simulink model "SG__MDL_IO104_setup"  (R2022a)
settings: Solver=FixedStepAuto  StartTime=0.0  StopTime=Inf  RelTol=1e-3  EnableMultiTasking=on
model workspace (MAT data in the model file):
  a = 0.28
  ff = 1200
  fi = 150
  tmax = 40
undefined symbols (not defined in the file or in its folder): Ended, Single
libraries: simulink x4, dspfdesign x3, speedgoatlib_IO104 x3, hdlsllib x2, slrealtimeloglib x1, dspsrcs4 x1
settings Model: SimulationMode=external  Creator=padlewsk  LastModifiedBy=padlewsk
settings SolverCC: ConcurrentTasks=on  AlgebraicLoopSolver=TrustRegion  PositivePriorityOrder=on  AutoInsertRateTranBlk=on
settings DataIOCC: SaveFormat=StructureWithTime
settings OptimizationCC: BlockReduction=off  OptimizeBlockIOStorage=off
settings DebuggingCC: TasksWithSamePriorityMsg=none  UnconnectedInputMsg=warning  UnconnectedOutputMsg=warning  UnconnectedLineMsg=warning
settings HardwareCC: ProdBitPerLong=64  ProdLongLongMode=on  ProdHWDeviceType=Intel->x86-64 (Linux 64)
settings RTWCC: Description=Simulink Real-Time  SystemTargetFile=slrealtime.tlc  TemplateMakefile=slrealtime_default_tmf  Toolchain=Simulink Real-Time Toolchain  BuildConfiguration=Faster Runs  CodeExecutionProfiling=on  TargetLang=C++

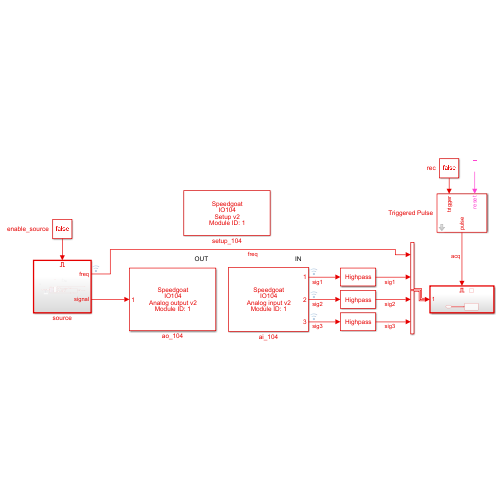
[thumbnail: Simulink's stored preview of the top-level diagram]
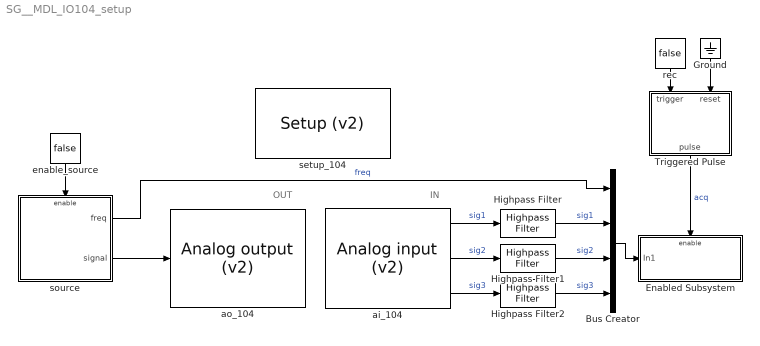
== system SG__MDL_IO104_setup ==
  note: IN
  note: OUT
  Bus Creator : BusCreator  Inputs=4
  Enabled Subsystem : Subsystem  TreatAsAtomicUnit=on
  Ground : Ground
  Highpass Filter : dspfdesign/Highpass Filter  FilterType=IIR  DesignForMinimumOrder=off  FilterOrder=4  StopbandFrequency=1  PassbandFrequency=5  StopbandAttenuation=40  PassbandRipple=0.5  InheritSampleRate=off  SampleRate=44100  SimulateUsing=Interpreted execution  roundingMode=Floor  coeffsDataTypeStr=fixdt(1,16)
  Highpass Filter1 : dspfdesign/Highpass Filter  FilterType=IIR  DesignForMinimumOrder=off  FilterOrder=4  StopbandFrequency=1  PassbandFrequency=5  StopbandAttenuation=40  PassbandRipple=0.5  InheritSampleRate=off  SampleRate=44100  SimulateUsing=Interpreted execution  roundingMode=Floor  coeffsDataTypeStr=fixdt(1,16)
  Highpass Filter2 : dspfdesign/Highpass Filter  FilterType=IIR  DesignForMinimumOrder=off  FilterOrder=4  StopbandFrequency=1  PassbandFrequency=5  StopbandAttenuation=40  PassbandRipple=0.5  InheritSampleRate=off  SampleRate=44100  SimulateUsing=Interpreted execution  roundingMode=Floor  coeffsDataTypeStr=fixdt(1,16)
  Triggered Pulse : Subsystem  mask(Triggered Pulse){N=4}
      mask prompts: N "Length (N samples)"
      mask help: Generates a single pulse of N samples length
  ai_104 : speedgoatlib_IO104/Analog input (v2)   parModuleId=1  parTs=0.0001  parPciSlot=-1  parAdChannels=[1,2,3]  parAdChannelsSorted=[1,2,3]  parAdRange1=+-2.5V  parAdRange2=+-2.5V  parAdCoupling=Single-Ended  parAdFrameSize=1  parAdUseTrigger=off  parAdClockInitiator=Initiator  parAdSampleTime=9.920634921e-07  parTriggerInitiator=Target  parTriggerRate=4.161015625e-01
      settings: SourceProductName=Simulink Real-Time: Speedgoat I/O Blockset
  ao_104 : speedgoatlib_IO104/Analog output (v2)   parModuleId=1  parTs=0.0001  parPciSlot=-1  parDaChannels=1  parDaChannelsSorted=1  parDaInitValue=0  parDaReset=1  parDaRange=+-2.5V  parDaFrameSize=1  parDaUseTrigger=off  parDaClockInitiator=Initiator  parDaSampleTime=9.920634921e-07  parTriggerInitiator=Target  parTriggerRate=4.161015625e-01  parAdBlockPresent=1
      settings: SourceProductName=Simulink Real-Time: Speedgoat I/O Blockset
  enable_source : Constant  Value=false  SampleTime=-1
  rec : Constant  Value=false  SampleTime=-1
  setup_104 : speedgoatlib_IO104/Setup (v2)   parPciSlot=-1  parModuleId=1  parTriggerInitiator=Target  parTriggerRate=4.161015625e-01  parCalibrate=off  parAdChannels=[1:3]  parAdRange1=+-2.5V  parAdRange2=+-2.5V  parAdCoupling=Single-Ended  parAdUseTrigger=off  parAdFrameSize=1  parAdClockInitiator=Initiator  parAdSampleTime=9.920634921e-07  parDaChannels=[1]  parDaChannelsSorted=1  parDaInitValue=[0]  parDaReset=[1]  parDaRange=+-2.5V  parDaUseTrigger=off  parDaFrameSize=1  parDaClockInitiator=Initiator  parDaSampleTime=9.920634921e-07  parDioByte0Dir=Outputs  parDioByte1Dir=Inputs  parDoChannels=[1:4]  parDoInitValues=[0]  parDoReset=[1]  parDiChannels=[13:16]
      settings: SourceProductName=Simulink Real-Time: Speedgoat I/O Blockset
  source : Subsystem  TreatAsAtomicUnit=on
  wires:
  enable_source/1 -> source/Enable
  source/2(signal) -> ao_104/1
  Triggered Pulse/1(pulse) -> Enabled Subsystem/Enable  "acq"
  Ground/1 -> Triggered Pulse/2(reset)
  rec/1 -> Triggered Pulse/1(trigger)
  Bus Creator/1 -> Enabled Subsystem/1(In1)
  source/1(freq) -> Bus Creator/1  "freq"
  ai_104/1 -> Highpass Filter/1  "sig1"
  ai_104/2 -> Highpass Filter1/1  "sig2"
  ai_104/3 -> Highpass Filter2/1  "sig3"
  Highpass Filter/1 -> Bus Creator/2  "sig1"
  Highpass Filter1/1 -> Bus Creator/3  "sig2"
  Highpass Filter2/1 -> Bus Creator/4  "sig3"

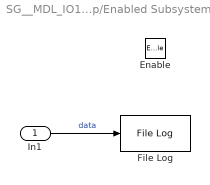
== system SG__MDL_IO104_setup/Enabled Subsystem ==
  In1 : Inport
  Enable : EnablePort
  File Log : slrealtimeloglib/File Log  decimation=1  inputProcessing=Elements as channels (sample based)
      settings: SourceProductBaseCode=XP
  wires:
  In1/1 -> File Log/1  "data"

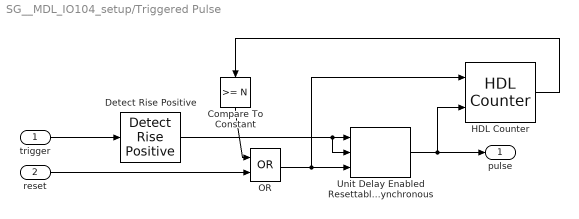
== system SG__MDL_IO104_setup/Triggered Pulse ==
  trigger : Inport
  reset : Inport  Port=2
  Compare To Constant : simulink/Logic and Bit Operations/Compare To Constant  relop=>=  const=N  OutDataTypeStr=boolean
  Detect Rise Positive : simulink/Logic and Bit Operations/Detect Rise Positive  vinit=0  OutDataTypeStr=boolean
  HDL Counter : hdlsllib/Sources/HDL Counter  CountType=Free running  CountInit=1  CountStep=1  CountMax=25  CountFromType=Initial value  CountFrom=1  CountResetPort=on  CountLoadPort=off  CountEnbPort=on  CountDirPort=off  CountHitOutputPort=off  CountDataType=Unsigned  CountWordLen=32  CountFracLen=0  CountSampTime=1
  OR : Logic  Operator=OR  AllPortsSameDT=off  OutDataTypeStr=boolean
  Unit Delay Enabled Resettable Synchronous : hdlsllib/Discrete/Unit Delay Enabled Resettable Synchronous  InitialCondition=0.0  SampleTime=-1
      settings: SourceProductBaseCode=SL
  pulse : Outport  VectorParamsAs1DForOutWhenUnconnected=off
  wires:
  OR/1 -> Unit Delay Enabled Resettable Synchronous/3, HDL Counter/1
  trigger/1 -> Detect Rise Positive/1
  Unit Delay Enabled Resettable Synchronous/1 -> HDL Counter/2, pulse/1
  Compare To Constant/1 -> OR/1
  reset/1 -> OR/2
  Detect Rise Positive/1 -> Unit Delay Enabled Resettable Synchronous/1, Unit Delay Enabled Resettable Synchronous/2
  HDL Counter/1 -> Compare To Constant/1

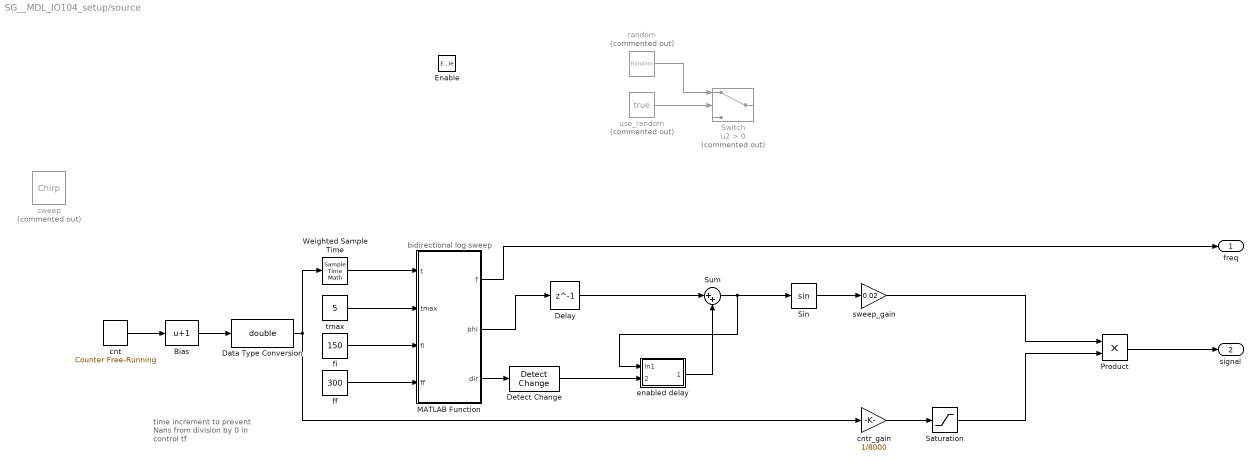
== system SG__MDL_IO104_setup/source ==
  note: bidirectional log sweep
  note: time increment to prevent Nans from division by 0 in control tf
  Enable : EnablePort  StatesWhenEnabling=reset
  Bias : Bias  Bias=1  SaturateOnIntegerOverflow=off
  Data Type Conversion : DataTypeConversion  OutDataTypeStr=double  SaturateOnIntegerOverflow=off  RndMeth=Floor
  Delay : Delay  DelayLength=1
  Detect Change : simulink/Logic and Bit Operations/Detect Change  vinit=false  OutDataTypeStr=boolean
  MATLAB Function : MATLAB Function  TreatAsAtomicUnit=on
  Product : Product
  Saturation : Saturate  UpperLimit=1  LowerLimit=0
  Sin : Trigonometry
  Sum : Sum  Inputs=|++
  Switch : Switch  Commented=on  Criteria=u2 > Threshold  SaturateOnIntegerOverflow=off  InputSameDT=off
  Weighted Sample Time : SampleTimeMath  TsampMathOp=*
  cnt : simulink/Sources/Counter Free-Running  NumBits=32  tsamp=-1
  cntr_gain : Gain  Gain=1/8000  ParamDataTypeStr=double
  enabled delay : Subsystem
  ff : Constant  Value=300
  fi : Constant  Value=150
  random : RandomNumber  Commented=on  Variance=0.5  SampleTime=3.5e-05
  sweep : dspsrcs4/Chirp  Commented=on  sweep=Logarithmic  mode=Bidirectional  f0=150  f1=1200  t1=10  Tsweep=20  phase=0  Ts=3.5e-05  spf=1  datatype=Double  OutputFrames=off
  sweep_gain : Gain  Gain=0.02
  tmax : Constant  Value=5
  use_random : Constant  Commented=on  Value=true  SampleTime=-1
  freq : Outport  OutputWhenDisabled=reset  InitialOutput=0  VectorParamsAs1DForOutWhenUnconnected=off
  signal : Outport  Port=2  OutputWhenDisabled=reset  InitialOutput=0  VectorParamsAs1DForOutWhenUnconnected=off
  wires:
  use_random/1 -> Switch/2
  random/1 -> Switch/1
  sweep_gain/1 -> Product/1
  cntr_gain/1 -> Saturation/1
  Product/1 -> signal/1
  MATLAB Function/2(phi) -> Delay/1
  Saturation/1 -> Product/2
  Weighted Sample Time/1 -> MATLAB Function/1(t)
  Data Type Conversion/1 -> cntr_gain/1, Weighted Sample Time/1
  MATLAB Function/1(f) -> freq/1
  Sin/1 -> sweep_gain/1
  MATLAB Function/3(dir) -> Detect Change/1
  Detect Change/1 -> enabled delay/2(enable)
  Delay/1 -> Sum/1
  enabled delay/1(Out1) -> Sum/2
  Sum/1 -> enabled delay/1(In1), Sin/1
  cnt/1 -> Bias/1
  Bias/1 -> Data Type Conversion/1
  ff/1 -> MATLAB Function/4(ff)
  tmax/1 -> MATLAB Function/2(tmax)
  fi/1 -> MATLAB Function/3(fi)

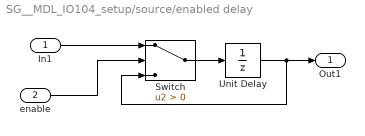
== system SG__MDL_IO104_setup/source/enabled delay ==
  In1 : Inport
  enable : Inport  Port=2
  Switch : Switch  Criteria=u2 > Threshold  SaturateOnIntegerOverflow=off  InputSameDT=off
  Unit Delay : UnitDelay  SampleTime=-1  HasFrameUpgradeWarning=on
  Out1 : Outport
  wires:
  Unit Delay/1 -> Switch/3, Out1/1
  Switch/1 -> Unit Delay/1
  In1/1 -> Switch/1
  enable/1 -> Switch/2

== matlab function SG__MDL_IO104_setup/source/MATLAB Function ==
  data: f output; t input; tmax input; phi output; dir output; fi input; ff input
function [f, phi, dir] = fcn(t, tmax, fi, ff)
%tmax is the time at which the maximum frequency is reached

t = mod(t, 2*tmax);

if t < tmax
    % up
    dir = 1;
    
    
    % linear (CF wikipedia)
%     phi = 2*pi*(0.5*(ff - fi)*t^2/tmax + fi*t);
%     f = fi + (ff - fi)*t/tmax;
    
    % logarithmic %%% https://en.wikipedia.org/wiki/Chirp
    k = log((ff/fi)^(1/tmax));
    phi = 2*pi*fi*(exp(k*t) - 1)/k;
    f = fi*exp(k*t);
else
    % down
    dir = -1;
    
    
    % linear (CF wikipedia)
%     phi = 2*pi*(0.5*(fi - ff)*(t-tmax)^2/tmax + ff*(t-tmax)); % linear
%     f = ff + (fi - ff)*(t - tmax)/tmax;
    
    % logarithmic
    k = log((fi/ff)^(1/tmax));
    phi = 2*pi*ff*(exp(k*(t - tmax)) - 1)/k;
    f = ff*exp(k*(t-tmax));
end

phi = mod(phi, 2*pi);
